simulink model "simu"  (R2024b)
settings: Solver=VariableStepAuto  StartTime=0.0  StopTime=45  RelTol=1e-3
undefined symbols (not defined in the file or in its folder): epsilon1, epsilon2, Km, Kx, Ky, n, T, theta0, waypoints, x0, y0
libraries: robotcorelib x1, mobileRoboticsLib x1
settings Model: Creator=Thibaud Piccinali  LastModifiedBy=Thibaud Piccinali

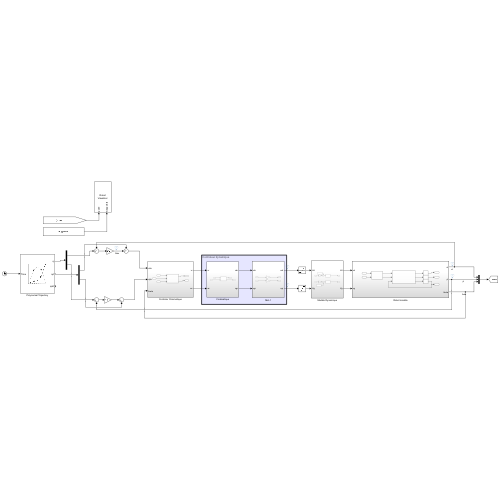
[thumbnail: Simulink's stored preview of the top-level diagram]
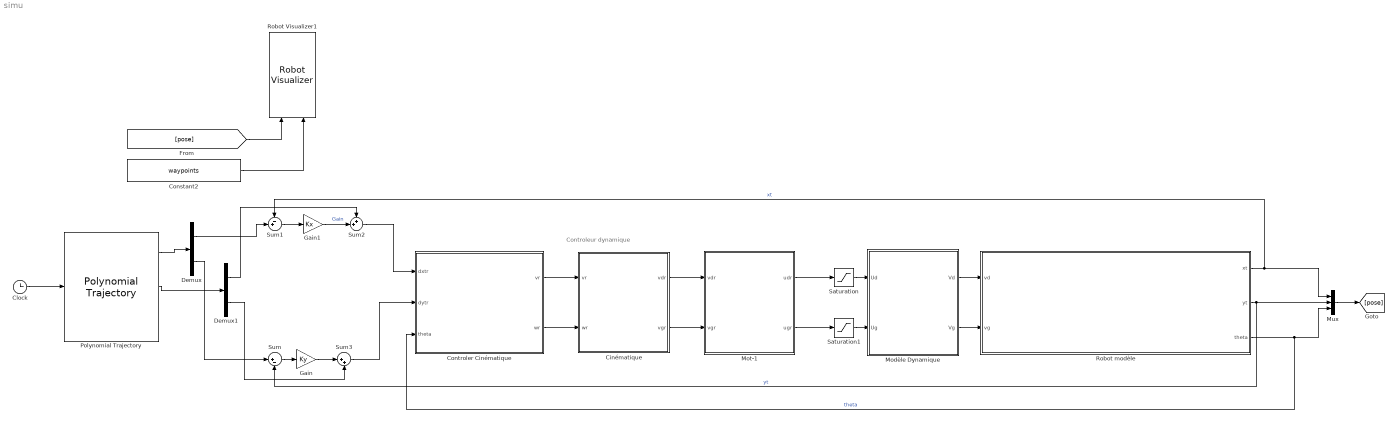
== system simu ==
  note: Controleur dynamique
  Cinématique : Subsystem
  Clock : Clock
  Constant2 : Constant  Value=waypoints
  Controler Cinématique : Subsystem
  Demux : Demux  Outputs=2
  Demux1 : Demux  Outputs=2
  Gain : Gain  Gain=Ky
  Gain1 : Gain  Gain=Kx
  Modèle Dynamique : Subsystem
  Mot-1 : Subsystem
  Mux : Mux  Inputs=3
  Polynomial Trajectory : robotcorelib/Polynomial Trajectory  WaypointSource=Internal  Waypoints=waypoints'  TimePoints=timepoints  TimeInterval=[ 1, 4 ]  Method=Cubic Polynomial  ParameterSource=Internal  VelocityBoundaryCondition=zeros(2,n)  AccelerationBoundaryCondition=zeros( 2, 5 )  SimulateUsing=Interpreted execution
  Robot Visualizer1 : mobileRoboticsLib/Environments/Robot Visualizer  robotRadius=0  mapName=entrepot  showTrajectory=on  hasWaypoints=on  hasLidar=off  sensorOffset=[ 0, 0 ]  scanAngles=[ -pi/4, 0, pi/4 ]  hasObjDetector=off  objDetectorOffset=[ 0, 0 ]  objDetectorAngle=0  objDetectorFOV=pi/4  objDetectorMaxRange=5  objectColors=[ 1, 0, 0; 0, 1, 0; 0, 0, 1 ]  objectMarkers=s
  Robot modèle : Subsystem
  Saturation : Saturate
  Saturation1 : Saturate
  Sum : Sum  Inputs=|+-
  Sum1 : Sum  Inputs=-+|
  Sum2 : Sum  Inputs=++|
  Sum3 : Sum  Inputs=|++
  wires:
  Mot-1/2(ugr) -> Saturation1/1
  Controler Cinématique/1(vr) -> Cinématique/1(vr)
  Saturation/1 -> Modèle Dynamique/1(Ud)
  Sum3/1 -> Controler Cinématique/2(dytr)
  Modèle Dynamique/2(Vg) -> Robot modèle/2(vg)
  Cinématique/2(vgr) -> Mot-1/2(vgr)
  Sum/1 -> Gain/1
  Gain1/1 -> Sum2/2  "Gain"
  Robot modèle/1(xt) -> Mux/1, Sum1/1  "xt"
  Robot modèle/3(theta) -> Controler Cinématique/3(theta), Mux/3  "theta"
  Robot modèle/2(yt) -> Sum/2, Mux/2  "yt"
  Controler Cinématique/2(wr) -> Cinématique/2(wr)
  Sum1/1 -> Gain1/1
  Sum2/1 -> Controler Cinématique/1(dxtr)
  Cinématique/1(vdr) -> Mot-1/1(vdr)
  Gain/1 -> Sum3/1
  Modèle Dynamique/1(Vd) -> Robot modèle/1(vd)
  Saturation1/1 -> Modèle Dynamique/2(Ug)
  Clock/1 -> Polynomial Trajectory/1
  Polynomial Trajectory/1 -> Demux/1
  Polynomial Trajectory/2 -> Demux1/1
  Demux/1 -> Sum1/2
  Demux1/1 -> Sum2/1
  Demux/2 -> Sum/1
  Demux1/2 -> Sum3/2
  Mux/1 -> [pose]
  [pose] -> Robot Visualizer1/1
  Constant2/1 -> Robot Visualizer1/2
  Mot-1/1(udr) -> Saturation/1

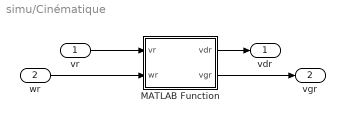
== system simu/Cinématique ==
  vr : Inport
  wr : Inport  Port=2
  MATLAB Function : MATLAB Function  TreatAsAtomicUnit=on
  vdr : Outport
  vgr : Outport  Port=2
  wires:
  vr/1 -> MATLAB Function/1(vr)
  wr/1 -> MATLAB Function/2(wr)
  MATLAB Function/1(vdr) -> vdr/1
  MATLAB Function/2(vgr) -> vgr/1

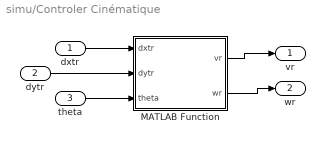
== system simu/Controler Cinématique ==
  dxtr : Inport
  dytr : Inport  Port=2
  theta : Inport  Port=3
  MATLAB Function : MATLAB Function  TreatAsAtomicUnit=on
  vr : Outport
  wr : Outport  Port=2
  wires:
  dxtr/1 -> MATLAB Function/1(dxtr)
  dytr/1 -> MATLAB Function/2(dytr)
  MATLAB Function/1(vr) -> vr/1
  MATLAB Function/2(wr) -> wr/1
  theta/1 -> MATLAB Function/3(theta)

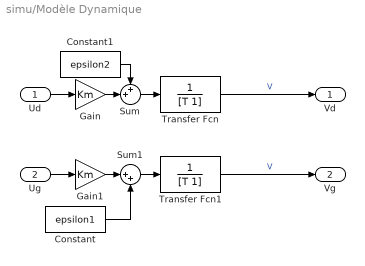
== system simu/Modèle Dynamique ==
  Ud : Inport
  Ug : Inport  Port=2
  Constant : Constant  Value=epsilon1
  Constant1 : Constant  Value=epsilon2
  Gain : Gain  Gain=Km
  Gain1 : Gain  Gain=Km
  Sum : Sum  Inputs=++|
  Sum1 : Sum  Inputs=|++
  Transfer Fcn : TransferFcn  Denominator=[T 1]
  Transfer Fcn1 : TransferFcn  Denominator=[T 1]
  Vd : Outport
  Vg : Outport  Port=2
  wires:
  Ug/1 -> Gain1/1
  Ud/1 -> Gain/1
  Transfer Fcn1/1 -> Vg/1  "V"
  Transfer Fcn/1 -> Vd/1  "V"
  Constant1/1 -> Sum/1
  Sum/1 -> Transfer Fcn/1
  Gain/1 -> Sum/2
  Gain1/1 -> Sum1/1
  Sum1/1 -> Transfer Fcn1/1
  Constant/1 -> Sum1/2

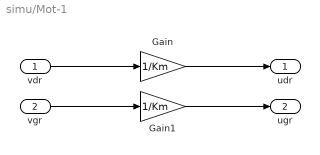
== system simu/Mot-1 ==
  vdr : Inport
  vgr : Inport  Port=2
  Gain : Gain  Gain=1/Km
  Gain1 : Gain  Gain=1/Km
  udr : Outport
  ugr : Outport  Port=2
  wires:
  vdr/1 -> Gain/1
  Gain/1 -> udr/1
  vgr/1 -> Gain1/1
  Gain1/1 -> ugr/1

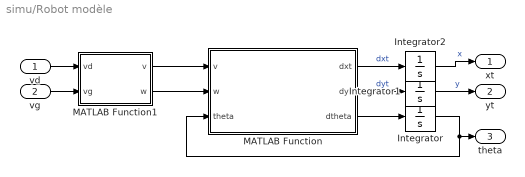
== system simu/Robot modèle ==
  vd : Inport
  vg : Inport  Port=2
  Integrator : Integrator  InitialCondition=theta0
  Integrator1 : Integrator  InitialCondition=y0
  Integrator2 : Integrator  InitialCondition=x0
  MATLAB Function : MATLAB Function  TreatAsAtomicUnit=on
  MATLAB Function1 : MATLAB Function  TreatAsAtomicUnit=on
  xt : Outport
  yt : Outport  Port=2
  theta : Outport  Port=3
  wires:
  MATLAB Function1/1(v) -> MATLAB Function/1(v)
  Integrator/1 -> theta/1, MATLAB Function/3(theta)
  MATLAB Function/3(dtheta) -> Integrator/1
  vg/1 -> MATLAB Function1/2(vg)
  MATLAB Function1/2(w) -> MATLAB Function/2(w)
  vd/1 -> MATLAB Function1/1(vd)
  Integrator2/1 -> xt/1  "x"
  Integrator1/1 -> yt/1  "y"
  MATLAB Function/1(dxt) -> Integrator2/1  "dxt"
  MATLAB Function/2(dyt) -> Integrator1/1  "dyt"

== matlab function simu/Robot modèle/MATLAB Function1 ==
  data: vd input; v output; vg input; w output; L parameter
function [v,w]= fcn(vd,vg,L)
 v = (vd+ vg)/2;
 w = (vd-vg)/(2*L);
end

== matlab function simu/Robot modèle/MATLAB Function ==
  data: dxt output; dyt output; v input; w input; dtheta output; theta input; L parameter
function [dxt,dyt,dtheta]= fcn(v,w,theta,L)
    dxt = cos(theta)*v - sin(theta)*L*w;
    dyt = sin(theta)*v + cos(theta)*L*w;
    dtheta = w;
end

== matlab function simu/Controler Cinématique/MATLAB Function ==
  data: dxtr input; vr output; dytr input; theta input; wr output; L parameter
function [vr,wr]= fcn(dxtr,dytr,theta,L)

vr = cos(theta)*dxtr + sin(theta)*dytr;
wr = (-sin(theta)*dxtr + cos(theta)*dytr)/L;

== matlab function simu/Cinématique/MATLAB Function ==
  data: vr input; vdr output; wr input; vgr output; l parameter
function [vdr,vgr]= fcn(vr,wr,l)
vdr = vr + l*wr;
vgr = vr - l*wr;
